simulink model "Estimations"  (R2023a)
settings: Solver=FixedStepAuto  StartTime=0.0  StopTime=150000  FixedStep=1  RelTol=1e-3
InitFcn:
  | load BatteryParameters.mat
values from neighbouring files (symbols this model uses):
  C1_LUT = [540 560 568 572 576 580 600 620 640 660 680 700 ... (105 elements, 21x5)]    [BatteryParameters.mat]
  Em_LUT = [3.147 3.292 3.392 3.477 3.518 3.561 3.602 3.638 3.677 3.719 3.763 3.799 ... (105 elements, 21x5)]    [BatteryParameters.mat]
  R1_LUT = [0.153117539 0.114898532 0.101253199 0.093222981 0.089962592 0.089117306 0.088090887 0.087366356 0.086883336 0.086038049 0.08477012 0.085313519 ... (105 elements, 21x5)]    [BatteryParameters.mat]
  SOC_LUT = [0 0.05 0.1 0.15 0.2 0.25 0.3 0.35 0.4 0.45 0.5 0.55 ... (21 elements, 21x1)]    [BatteryParameters.mat]
  Temperature_LUT = [263.15 273.15 298.15 318.15 333.15]    [BatteryParameters.mat]
  Ts = 1    [BatteryParameters.mat]
libraries: sharedTrackingLibrary x9
(part 2 of 2)

== system Estimations/Subsystem6/Simulink Function - State Transition Function1 ==
  Current : Inport
  Temperature (K) : Inport  Port=2
  Estimated Cq : Inport  Port=3
  batteryStateFcn6 : TriggerPort  TriggerType=function-call  IsSimulinkFunction=on  FunctionName=batteryStateFcn6  VariantControl=Variant
  Add : Sum
  C1 Table : Lookup_n-D  BreakpointsForDimension1=SOC_LUT  BreakpointsForDimension2=Temperature_LUT  Table=C1_LUT  InternalRulePriority=Speed  RndMeth=Simplest
      settings: InputPortMap=u0,u1
  Constant : Constant  Value=Ts
  Get SOC : Selector  InputPortWidth=3  IndexOptions=Index vector (dialog)  Indices=1  OutputSizes=1
  Product : Product
  R1 Table : Lookup_n-D  BreakpointsForDimension1=SOC_LUT  BreakpointsForDimension2=Temperature_LUT  Table=R1_LUT  InternalRulePriority=Speed  RndMeth=Simplest
      settings: InputPortMap=u0,u1
  f(x,u) : MATLAB Function  TreatAsAtomicUnit=on
  x1 : ArgIn  DisableCoverage=on  PortDimensions=3  ArgumentName=x1
  x1Next : ArgOut  DisableCoverage=on  PortDimensions=3  ArgumentName=x1Next
  wires:
  Estimated Cq/1 -> f(x,u)/4(Cq)
  Product/1 -> Add/2
  f(x,u)/1(xdot) -> Product/1
  Constant/1 -> Product/2
  Current/1 -> f(x,u)/5(I)
  R1 Table/1 -> f(x,u)/3(R1)
  C1 Table/1 -> f(x,u)/2(C1)
  Get SOC/1 -> C1 Table/1, R1 Table/1
  Temperature (K)/1 -> C1 Table/2, R1 Table/2
  Add/1 -> x1Next/1
  x1/1 -> Get SOC/1, Add/1, f(x,u)/1(x)

== system Estimations/Subsystem7/Simulink Function - Measurement Function1 ==
  Current : Inport
  Temperature (K) : Inport  Port=2
  batteryMeasurementFcn7 : TriggerPort  TriggerType=function-call  IsSimulinkFunction=on  FunctionName=batteryMeasurementFcn7  VariantControl=Variant
  Add1 : Sum  Inputs=+--
  Em Table : Lookup_n-D  BreakpointsForDimension1=SOC_LUT  BreakpointsForDimension2=Temperature_LUT  Table=Em_LUT  InternalRulePriority=Speed  RndMeth=Simplest
      settings: InputPortMap=u0,u1
  Get SOC : Selector  InputPortWidth=3  IndexOptions=Index vector (dialog)  Indices=[1]  OutputSizes=1
  Get U1 : Selector  InputPortWidth=3  IndexOptions=Index vector (dialog)  Indices=2  OutputSizes=1
  Get U2 : Selector  InputPortWidth=3  IndexOptions=Index vector (dialog)  Indices=3  OutputSizes=1
  Product : Product
  x1 : ArgIn  DisableCoverage=on  PortDimensions=3  ArgumentName=x1
  y1 : ArgOut  DisableCoverage=on  ArgumentName=y1
  wires:
  x1/1 -> Get U1/1, Get U2/1, Get SOC/1
  Get SOC/1 -> Em Table/1  "SOC"
  Em Table/1 -> Add1/1
  Add1/1 -> y1/1
  Temperature (K)/1 -> Em Table/2
  Get U2/1 -> Product/1
  Current/1 -> Product/2
  Product/1 -> Add1/2
  Get U1/1 -> Add1/3  "U1"

== system Estimations/Subsystem7/Simulink Function - State Transition Function1 ==
  Current : Inport
  Temperature (K) : Inport  Port=2
  Estimated Cq : Inport  Port=3
  batteryStateFcn7 : TriggerPort  TriggerType=function-call  IsSimulinkFunction=on  FunctionName=batteryStateFcn7  VariantControl=Variant
  Add : Sum
  C1 Table : Lookup_n-D  BreakpointsForDimension1=SOC_LUT  BreakpointsForDimension2=Temperature_LUT  Table=C1_LUT  InternalRulePriority=Speed  RndMeth=Simplest
      settings: InputPortMap=u0,u1
  Constant : Constant  Value=Ts
  Get SOC : Selector  InputPortWidth=3  IndexOptions=Index vector (dialog)  Indices=1  OutputSizes=1
  Product : Product
  R1 Table : Lookup_n-D  BreakpointsForDimension1=SOC_LUT  BreakpointsForDimension2=Temperature_LUT  Table=R1_LUT  InternalRulePriority=Speed  RndMeth=Simplest
      settings: InputPortMap=u0,u1
  f(x,u) : MATLAB Function  TreatAsAtomicUnit=on
  x1 : ArgIn  DisableCoverage=on  PortDimensions=3  ArgumentName=x1
  x1Next : ArgOut  DisableCoverage=on  PortDimensions=3  ArgumentName=x1Next
  wires:
  x1/1 -> f(x,u)/1(x), Add/1, Get SOC/1
  Add/1 -> x1Next/1
  Temperature (K)/1 -> R1 Table/2, C1 Table/2
  Get SOC/1 -> R1 Table/1, C1 Table/1
  C1 Table/1 -> f(x,u)/2(C1)
  R1 Table/1 -> f(x,u)/3(R1)
  Current/1 -> f(x,u)/5(I)
  Constant/1 -> Product/2
  f(x,u)/1(xdot) -> Product/1
  Product/1 -> Add/2
  Estimated Cq/1 -> f(x,u)/4(Cq)

== system Estimations/Subsystem8/Simulink Function - Measurement Function1 ==
  Current : Inport
  Temperature (K) : Inport  Port=2
  batteryMeasurementFcn8 : TriggerPort  TriggerType=function-call  IsSimulinkFunction=on  FunctionName=batteryMeasurementFcn8  VariantControl=Variant
  Add1 : Sum  Inputs=+--
  Em Table : Lookup_n-D  BreakpointsForDimension1=SOC_LUT  BreakpointsForDimension2=Temperature_LUT  Table=Em_LUT  InternalRulePriority=Speed  RndMeth=Simplest
      settings: InputPortMap=u0,u1
  Get SOC : Selector  InputPortWidth=3  IndexOptions=Index vector (dialog)  Indices=[1]  OutputSizes=1
  Get U1 : Selector  InputPortWidth=3  IndexOptions=Index vector (dialog)  Indices=2  OutputSizes=1
  Get U2 : Selector  InputPortWidth=3  IndexOptions=Index vector (dialog)  Indices=3  OutputSizes=1
  Product : Product
  x1 : ArgIn  DisableCoverage=on  PortDimensions=3  ArgumentName=x1
  y1 : ArgOut  DisableCoverage=on  ArgumentName=y1
  wires:
  Get U1/1 -> Add1/3  "U1"
  Product/1 -> Add1/2
  Current/1 -> Product/2
  Get U2/1 -> Product/1
  Temperature (K)/1 -> Em Table/2
  Add1/1 -> y1/1
  Em Table/1 -> Add1/1
  Get SOC/1 -> Em Table/1  "SOC"
  x1/1 -> Get SOC/1, Get U2/1, Get U1/1

== system Estimations/Subsystem8/Simulink Function - State Transition Function1 ==
  Current : Inport
  Temperature (K) : Inport  Port=2
  Estimated Cq : Inport  Port=3
  batteryStateFcn8 : TriggerPort  TriggerType=function-call  IsSimulinkFunction=on  FunctionName=batteryStateFcn8  VariantControl=Variant
  Add : Sum
  C1 Table : Lookup_n-D  BreakpointsForDimension1=SOC_LUT  BreakpointsForDimension2=Temperature_LUT  Table=C1_LUT  InternalRulePriority=Speed  RndMeth=Simplest
      settings: InputPortMap=u0,u1
  Constant : Constant  Value=Ts
  Get SOC : Selector  InputPortWidth=3  IndexOptions=Index vector (dialog)  Indices=1  OutputSizes=1
  Product : Product
  R1 Table : Lookup_n-D  BreakpointsForDimension1=SOC_LUT  BreakpointsForDimension2=Temperature_LUT  Table=R1_LUT  InternalRulePriority=Speed  RndMeth=Simplest
      settings: InputPortMap=u0,u1
  f(x,u) : MATLAB Function  TreatAsAtomicUnit=on
  x1 : ArgIn  DisableCoverage=on  PortDimensions=3  ArgumentName=x1
  x1Next : ArgOut  DisableCoverage=on  PortDimensions=3  ArgumentName=x1Next
  wires:
  Estimated Cq/1 -> f(x,u)/4(Cq)
  Product/1 -> Add/2
  f(x,u)/1(xdot) -> Product/1
  Constant/1 -> Product/2
  Current/1 -> f(x,u)/5(I)
  R1 Table/1 -> f(x,u)/3(R1)
  C1 Table/1 -> f(x,u)/2(C1)
  Get SOC/1 -> C1 Table/1, R1 Table/1
  Temperature (K)/1 -> C1 Table/2, R1 Table/2
  Add/1 -> x1Next/1
  x1/1 -> Get SOC/1, Add/1, f(x,u)/1(x)

== system Estimations/Subsystem9/Simulink Function - Measurement Function1 ==
  Current : Inport
  Temperature (K) : Inport  Port=2
  batteryMeasurementFcn9 : TriggerPort  TriggerType=function-call  IsSimulinkFunction=on  FunctionName=batteryMeasurementFcn9  VariantControl=Variant
  Add1 : Sum  Inputs=+--
  Em Table : Lookup_n-D  BreakpointsForDimension1=SOC_LUT  BreakpointsForDimension2=Temperature_LUT  Table=Em_LUT  InternalRulePriority=Speed  RndMeth=Simplest
      settings: InputPortMap=u0,u1
  Get SOC : Selector  InputPortWidth=3  IndexOptions=Index vector (dialog)  Indices=[1]  OutputSizes=1
  Get U1 : Selector  InputPortWidth=3  IndexOptions=Index vector (dialog)  Indices=2  OutputSizes=1
  Get U2 : Selector  InputPortWidth=3  IndexOptions=Index vector (dialog)  Indices=3  OutputSizes=1
  Product : Product
  x1 : ArgIn  DisableCoverage=on  PortDimensions=3  ArgumentName=x1
  y1 : ArgOut  DisableCoverage=on  ArgumentName=y1
  wires:
  x1/1 -> Get U1/1, Get U2/1, Get SOC/1
  Get SOC/1 -> Em Table/1  "SOC"
  Em Table/1 -> Add1/1
  Add1/1 -> y1/1
  Temperature (K)/1 -> Em Table/2
  Get U2/1 -> Product/1
  Current/1 -> Product/2
  Product/1 -> Add1/2
  Get U1/1 -> Add1/3  "U1"

== system Estimations/Subsystem9/Simulink Function - State Transition Function1 ==
  Current : Inport
  Temperature (K) : Inport  Port=2
  Estimated Cq : Inport  Port=3
  batteryStateFcn9 : TriggerPort  TriggerType=function-call  IsSimulinkFunction=on  FunctionName=batteryStateFcn9  VariantControl=Variant
  Add : Sum
  C1 Table : Lookup_n-D  BreakpointsForDimension1=SOC_LUT  BreakpointsForDimension2=Temperature_LUT  Table=C1_LUT  InternalRulePriority=Speed  RndMeth=Simplest
      settings: InputPortMap=u0,u1
  Constant : Constant  Value=Ts
  Get SOC : Selector  InputPortWidth=3  IndexOptions=Index vector (dialog)  Indices=1  OutputSizes=1
  Product : Product
  R1 Table : Lookup_n-D  BreakpointsForDimension1=SOC_LUT  BreakpointsForDimension2=Temperature_LUT  Table=R1_LUT  InternalRulePriority=Speed  RndMeth=Simplest
      settings: InputPortMap=u0,u1
  f(x,u) : MATLAB Function  TreatAsAtomicUnit=on
  x1 : ArgIn  DisableCoverage=on  PortDimensions=3  ArgumentName=x1
  x1Next : ArgOut  DisableCoverage=on  PortDimensions=3  ArgumentName=x1Next
  wires:
  x1/1 -> f(x,u)/1(x), Add/1, Get SOC/1
  Add/1 -> x1Next/1
  Temperature (K)/1 -> R1 Table/2, C1 Table/2
  Get SOC/1 -> R1 Table/1, C1 Table/1
  C1 Table/1 -> f(x,u)/2(C1)
  R1 Table/1 -> f(x,u)/3(R1)
  Current/1 -> f(x,u)/5(I)
  Constant/1 -> Product/2
  f(x,u)/1(xdot) -> Product/1
  Product/1 -> Add/2
  Estimated Cq/1 -> f(x,u)/4(Cq)

== matlab function Estimations/Subsystem9/Simulink Function - State Transition Function1/f(x,u) ==
  data: x input; C1 input; R1 input; Cq input; I input; xdot output
function xdot = fx(x,C1,R1,Cq,I)
xdot = zeros(size(x));
U1 = x(2);
xdot(1) = -I/(3600*Cq);
xdot(2) = -1/(R1*C1)*U1 + I/C1;
xdot(3) = 0;

== matlab function Estimations/Subsystem1/Simulink Function - State Transition Function1/f(x,u) ==
  data: x input; C1 input; R1 input; Cq input; I input; xdot output
function xdot = fx(x,C1,R1,Cq,I)
xdot = zeros(size(x));
U1 = x(2);
xdot(1) = -I/(3600*Cq);
xdot(2) = -1/(R1*C1)*U1 + I/C1;
xdot(3) = 0;

== matlab function Estimations/Subsystem2/Simulink Function - State Transition Function2/f(x,u) ==
  data: x input; C1 input; R1 input; Cq input; I input; xdot output
function xdot = fx(x,C1,R1,Cq,I)
xdot = zeros(size(x));
U1 = x(2);
xdot(1) = -I/(3600*Cq);
xdot(2) = -1/(R1*C1)*U1 + I/C1;
xdot(3) = 0;

== matlab function Estimations/Subsystem3/Simulink Function - State Transition Function1/f(x,u) ==
  data: x input; C1 input; R1 input; Cq input; I input; xdot output
function xdot = fx(x,C1,R1,Cq,I)
xdot = zeros(size(x));
U1 = x(2);
xdot(1) = -I/(3600*Cq);
xdot(2) = -1/(R1*C1)*U1 + I/C1;
xdot(3) = 0;

== matlab function Estimations/Subsystem4/Simulink Function - State Transition Function1/f(x,u) ==
  data: x input; C1 input; R1 input; Cq input; I input; xdot output
function xdot = fx(x,C1,R1,Cq,I)
xdot = zeros(size(x));
U1 = x(2);
xdot(1) = -I/(3600*Cq);
xdot(2) = -1/(R1*C1)*U1 + I/C1;
xdot(3) = 0;

== matlab function Estimations/Subsystem5/Simulink Function - State Transition Function1/f(x,u) ==
  data: x input; C1 input; R1 input; Cq input; I input; xdot output
function xdot = fx(x,C1,R1,Cq,I)
xdot = zeros(size(x));
U1 = x(2);
xdot(1) = -I/(3600*Cq);
xdot(2) = -1/(R1*C1)*U1 + I/C1;
xdot(3) = 0;

== matlab function Estimations/Subsystem6/Simulink Function - State Transition Function1/f(x,u) ==
  data: x input; C1 input; R1 input; Cq input; I input; xdot output
function xdot = fx(x,C1,R1,Cq,I)
xdot = zeros(size(x));
U1 = x(2);
xdot(1) = -I/(3600*Cq);
xdot(2) = -1/(R1*C1)*U1 + I/C1;
xdot(3) = 0;

== matlab function Estimations/Subsystem7/Simulink Function - State Transition Function1/f(x,u) ==
  data: x input; C1 input; R1 input; Cq input; I input; xdot output
function xdot = fx(x,C1,R1,Cq,I)
xdot = zeros(size(x));
U1 = x(2);
xdot(1) = -I/(3600*Cq);
xdot(2) = -1/(R1*C1)*U1 + I/C1;
xdot(3) = 0;

== matlab function Estimations/Subsystem8/Simulink Function - State Transition Function1/f(x,u) ==
  data: x input; C1 input; R1 input; Cq input; I input; xdot output
function xdot = fx(x,C1,R1,Cq,I)
xdot = zeros(size(x));
U1 = x(2);
xdot(1) = -I/(3600*Cq);
xdot(2) = -1/(R1*C1)*U1 + I/C1;
xdot(3) = 0;
